simulink model "OPSGC"  (R2023a)
settings: Solver=VariableStepAuto  StartTime=0.0  StopTime=5  RelTol=1e-3
values from neighbouring files (symbols this model uses):
  Kd = diag([150,150,150,20,20,20])    [parameters.m]
  Kp = diag([200,200,200,50,50,50])    [parameters.m]
  xd = [H(1:3,4); eulers']    [parameters.m]
settings Model: Creator=uzair  LastModifiedBy=syedj
settings OptimizationCC: ReuseModelBlockBuffer=off

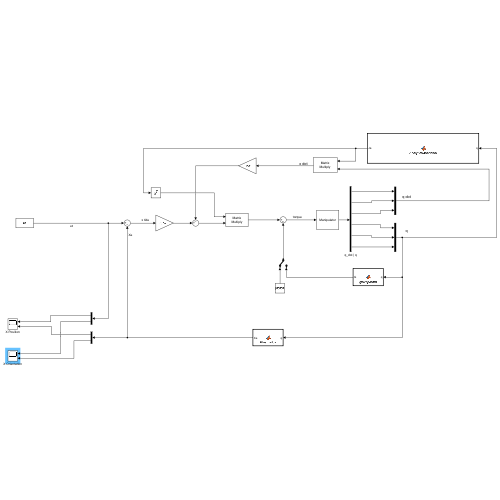
[thumbnail: Simulink's stored preview of the top-level diagram]
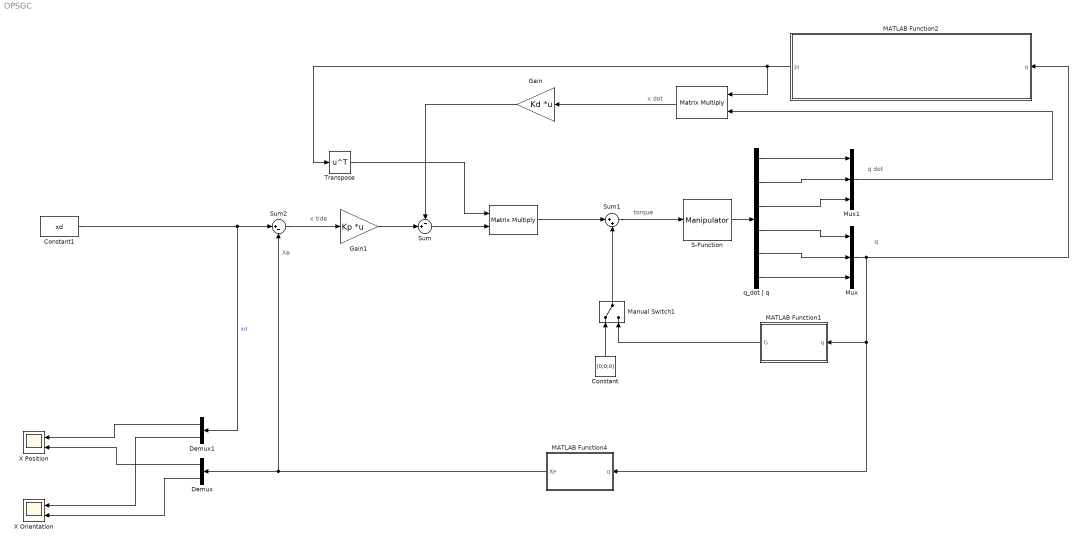
== system OPSGC ==
  note: torque
  note: x tide
  note: q
  note: q dot
  note: Xe
  note: x dot
  " " : Product  Multiplication=Matrix(*)
  "  " : Product  Multiplication=Matrix(*)
  Constant : Constant  Value=[0;0;0]
  Constant1 : Constant  Value=xd
  Demux : Demux  Outputs=2
  Demux1 : Demux  Outputs=2
  Gain : Gain  Gain=Kd  Multiplication=Matrix(K*u)
  Gain1 : Gain  Gain=Kp  Multiplication=Matrix(K*u)
  MATLAB Function1 : MATLAB Function  TreatAsAtomicUnit=on
  MATLAB Function2 : MATLAB Function  TreatAsAtomicUnit=on
  MATLAB Function4 : MATLAB Function  TreatAsAtomicUnit=on
  Manual Switch1 : ManualSwitch
  Mux : Mux  Inputs=3
  Mux1 : Mux  Inputs=3
  S-Function : S-Function  FunctionName=Manipulator  Parameters=params  SFunctionDeploymentMode=off  EnableBusSupport=off
  Sum : Sum  Inputs=-+|
  Sum1 : Sum  Inputs=|++
  Sum2 : Sum  Inputs=|+-
  Transpose : Math  Operator=transpose
  X Orientation : Scope  NumInputPorts=2
  X Position : Scope  NumInputPorts=2
  q_dot | q : Demux  Outputs=6
  wires:
  S-Function/1 -> q_dot | q/1
  q_dot | q/6 -> Mux/3
  q_dot | q/5 -> Mux/2
  q_dot | q/4 -> Mux/1
  q_dot | q/1 -> Mux1/1
  q_dot | q/2 -> Mux1/2
  q_dot | q/3 -> Mux1/3
  Gain/1 -> Sum/1
  Sum1/1 -> S-Function/1
  Mux/1 -> MATLAB Function2/1(q), MATLAB Function1/1(q), MATLAB Function4/1(q)
  Sum2/1 -> Gain1/1
  MATLAB Function1/1(G) -> Manual Switch1/2
  Constant/1 -> Manual Switch1/1
  Mux1/1 -> "  "/2
  MATLAB Function4/1(Xe) -> Demux/1, Sum2/2
  Constant1/1 -> Demux1/1, Sum2/1  "xd"
  Demux1/1 -> X Position/1
  Demux/1 -> X Position/2
  Demux1/2 -> X Orientation/1
  Demux/2 -> X Orientation/2
  Manual Switch1/1 -> Sum1/2
  MATLAB Function2/1(Ja) -> "  "/1, Transpose/1
  "  "/1 -> Gain/1
  Transpose/1 -> " "/1
  " "/1 -> Sum1/1
  Gain1/1 -> Sum/2
  Sum/1 -> " "/2

== matlab function OPSGC/MATLAB Function1 ==
  data: q input; G output; params parameter
function G = gravityMatrix(q, params)
    q1 = q(1);
    q2 = q(2);
    q3 = q(3);
    
    g = params.g;

    m1 = params.m(1);
    m2 = params.m(2);
    m3 = params.m(3);

    a1 = 0.02;
    a2 = 0.03;
    a3 = 0.01;
    b1 = 0.1256;
    b2 = 0.03;
    b3 = 0.01;
    c1 = 0.4;
    c2 = 0.46;
    c3 = 0.15;

    G = [(c1*g*m1*cos(q1))/2 + g*m2*cos(q1)*(c1 - c2/2) + g*m3*cos(q1)*(c1 + c3/2 + q3)
        0;
        g*m3*sin(q1)];
    
end

== matlab function OPSGC/MATLAB Function2 ==
  data: q input; Ja output
function Ja = AnalyticalJacobian(q)
    q1 = q(1);
    q2 = q(2);
    q3 = q(3);

    r1 = 0.4;
    a1 = 0.02;
    a2 = 0.03;
    a3 = 0.01;
    b1 = 0.1256;
    b2 = 0.03;
    b3 = 0.01;
    c1 = 0.4;
    c2 = 0.46;
    c3 = 0.15;

    H = [[0, -sin(q1), cos(q1),              cos(q1)*(c1 + c3 + q3)]
[1,        0,       0,                           - c2 - q2]
[0,  cos(q1), sin(q1), r1 + sin(q1)*(c3 + q3) + c1*sin(q1)]
[0,        0,       0,                                   1]];


eulers = rotm2eul(H(1:3,1:3), "ZYZ");


    phi1 = eulers(1);
    phi2 = eulers(2);
    phi3 = eulers(3);
    a1 = 0.02;
    a2 = 0.03;
    a3 = 0.01;
    b1 = 0.1256;
    b2 = 0.03;
    b3 = 0.01;
    c1 = 0.4;
    c2 = 0.46;
    c3 = 0.15;

Ja_m = [
[        -sin(q1)*(c1 + c3 + q3),  0, cos(q1)]
[                              0, -1,       0]
[         cos(q1)*(c1 + c3 + q3),  0, sin(q1)]
[(cos(phi2)*sin(phi1))/sin(phi2),  0,       0]
[                     -cos(phi1),  0,       0]
[           -sin(phi1)/sin(phi2),  0,       0]
];


    Ja = Ja_m;
end

== matlab function OPSGC/MATLAB Function4 ==
  data: q input; Xe output
function Xe = Kinematics(q)
    q1 = q(1);
    q2 = q(2);
    q3 = q(3);

    r1 = 0.4;
    a1 = 0.02;
    a2 = 0.03;
    a3 = 0.01;
    b1 = 0.1256;
    b2 = 0.03;
    b3 = 0.01;
    c1 = 0.4;
    c2 = 0.46;
    c3 = 0.15;
    
    H = [[0, -sin(q1), cos(q1),              cos(q1)*(c1 + c3 + q3)]
[1,        0,       0,                           - c2 - q2]
[0,  cos(q1), sin(q1), r1 + sin(q1)*(c3 + q3) + c1*sin(q1)]
[0,        0,       0,                                   1]
];

    eulers = rotm2eul(H(1:3,1:3), "ZYZ");

    Xe = [H(1:3,4); eulers'];
end
